simulink model "Robot_control"  (R2020b)
settings: Solver=FixedStepAuto  StartTime=0.0  StopTime=inf  FixedStep=0.01  RelTol=1e-3
values from neighbouring files (symbols this model uses):
  Initial_pos = [20 20 10]    [Robot_control_script.m]
  min_pwm_change = 0.39    [Robot_control_script.m]
  Motorspeed_MG996 = 60/.17    (= 352.941176471)    [Robot_control_script.m]
  Time_to_wait = [1 10]    [Robot_control_script.m]
  weights = [1 1 1 1 1 1]    [Robot_control_script.m]
undefined symbols (not defined in the file or in its folder): DiscIntNeverNeededParam, Levenberg, Marquardt, read_the_data, send_serial, Serial_Port, Standard_Devices
libraries: sldrtlib x4, simulink x3, robotcorelib x2, robotmaniplib x1, simulink_extras x1, dspstat3 x1, mspfiltlib x1, dspfdesign x1
(part 2 of 2)

== matlab function Robot_control/Ver 2.0 Haptic Robot Control/Motor Driver System/Orien Processing/Kalman and AHRS/MATLAB Function ==
  data: accRawX input; accAngleX output; accAngleY output; accRawY input; accRawZ input; accAngleZ output
function [accAngleX, accAngleY, accAngleZ] = fcn(accRawX, accRawY, accRawZ)

%Converting the raw accel data from g values to accel about X and Y axis

accAngleX = atan(accRawY/sqrt(power(accRawX,2) + power(accRawZ,2)))*(180/pi);
accAngleY = atan(-1*(accRawX/sqrt(power(accRawY,2) + power(accRawZ,2))))*(180/pi);
accAngleZ = atan(accRawZ/sqrt(power(accRawX,2) + power(accRawZ,2)))*(180/pi);

end
